simulink subsystem "edge1x1_asSubsystem"  (R2021a)
settings: Solver=VariableStepAuto  StartTime=0.0  StopTime=10.0  RelTol=1e-3
libraries: simulink x1
settings Model: Creator=phill  LastModifiedBy=phill

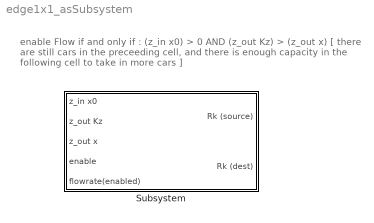
== system edge1x1_asSubsystem ==
  note: enable Flow if and only if : (z_in x0) > 0 AND (z_out Kz) > (z_out x)
      | [ there are still cars in the preceeding cell, and there is enough capacity
      | in the following cell to take in more cars ]
  Subsystem : Subsystem
      mask help: This block serves to establish a flow between two Street Lane Segments. To archieve this, it connects one source-cell [z_in] to one destination-cell [z_out], and prompts a flow of cars with the flowrate 'flowrate(enabled)' (an input) if and only if there are still cars at the end of [z_out] avaiable AND if the capacity of [z_out] is not yet surpassed, i.e. (z_in x0 > 0 AND z_out Kz > z_out x), AND if the 'enable' input is set to 1, otherwise the flow is reduced to 0.
      mask Display: disp('Edge 1x1');

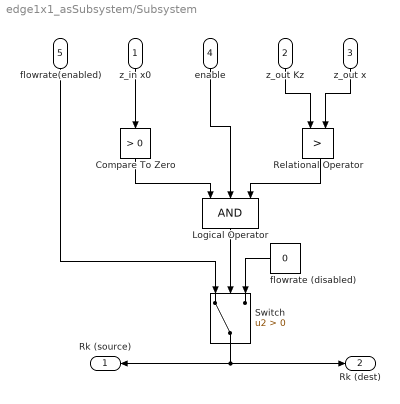
== system edge1x1_asSubsystem/Subsystem ==
  z_in x0 : Inport
  z_out Kz : Inport  Port=2
  z_out x : Inport  Port=3
  enable : Inport  Port=4
  flowrate(enabled) : Inport  Port=5
  Compare To Zero : simulink/Logic and Bit Operations/Compare To Zero  relop=>  OutDataTypeStr=boolean
  Logical Operator : Logic  Inputs=3  AllPortsSameDT=off  OutDataTypeStr=boolean
  Relational Operator : RelationalOperator  Operator=>  OutDataTypeStr=boolean  RndMeth=Simplest
  Switch : Switch  Criteria=u2 > Threshold
  flowrate (disabled) : Constant  Value=0
  Rk (source) : Outport
  Rk (dest) : Outport  Port=2
  wires:
  Switch/1 -> Rk (dest)/1, Rk (source)/1
  Relational Operator/1 -> Logical Operator/3
  Compare To Zero/1 -> Logical Operator/1
  z_in x0/1 -> Compare To Zero/1
  flowrate (disabled)/1 -> Switch/3
  flowrate(enabled)/1 -> Switch/1
  Logical Operator/1 -> Switch/2
  z_out x/1 -> Relational Operator/2
  enable/1 -> Logical Operator/2
  z_out Kz/1 -> Relational Operator/1
